simulink model "Simulink_Lin_og_NonLin"  (R2020b)
settings: Solver=VariableStepAuto  StartTime=0.0  StopTime=4  RelTol=1e-3
values from neighbouring files (symbols this model uses):
  b = 0.1    [Simulink_konstanter.m]
  g = 9.82    [Simulink_konstanter.m]
  I = 1/12    (= 0.0833333333333)    [Simulink_konstanter.m]
  Kp = 30    [Simulink_konstanter.m]
  l = 0.5    [Simulink_konstanter.m]
  m = 1    [Simulink_konstanter.m]
  Td = 1/7    (= 0.142857142857)    [Simulink_konstanter.m]
  Ti = 1    [Simulink_konstanter.m]
  u_bar = -(l*g*m*sqrt(3)) / 2    [Simulink_konstanter.m]
  y_bar = pi/3    (= 1.0471975512)    [Simulink_konstanter.m]
settings Model: Creator=madsw  LastModifiedBy=madsw

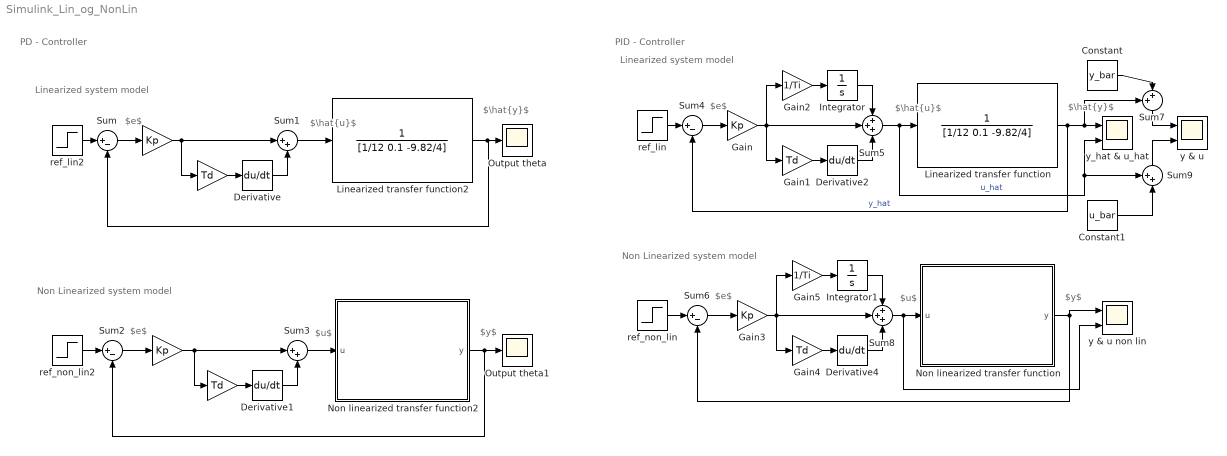
== system Simulink_Lin_og_NonLin ==
  note: PD - Controller
  note: Linearized system model
  note: Non Linearized system model
  note: $\hat{u}$
  note: $\hat{y}$
  note: $e$
  note: $u$
  note: $y$
  note: $e$
  note: Non Linearized system model
  note: $u$
  note: $y$
  note: Linearized system model
  note: $e$
  note: $\hat{u}$
  note: $\hat{y}$
  note: $e$
  note: PID - Controller
  " " : Gain  Gain=Td
  "  " : Gain  Gain=Kp
  "     " : Gain  Gain=Kp
  "              " : Gain  Gain=Td
  Constant : Constant  Value=y_bar
  Constant1 : Constant  Value=u_bar
  Derivative{,1..2,4} (4 alike) : Derivative
  Gain : Gain  Gain=Kp
  Gain1 : Gain  Gain=Td
  Gain2 : Gain  Gain=1/Ti
  Gain3 : Gain  Gain=Kp
  Gain4 : Gain  Gain=Td
  Gain5 : Gain  Gain=1/Ti
  Integrator : Integrator
  Integrator1 : Integrator
  Linearized transfer function : TransferFcn  Numerator=1  Denominator=[1/12 0.1 -9.82/4]
  Linearized transfer function2 : TransferFcn  Numerator=1  Denominator=[1/12 0.1 -9.82/4]
  Non linearized transfer function : Subsystem
  Non linearized transfer function2 : Subsystem
  Output theta : Scope
  Output theta1 : Scope
  Sum{,2,4,6} (4 alike) : Sum  Inputs=|+-
  Sum1 : Sum  Inputs=|++
  Sum3 : Sum  Inputs=|++
  Sum5 : Sum  Inputs=+++
  Sum7 : Sum  Inputs=++|
  Sum8 : Sum  Inputs=+++
  Sum9 : Sum  Inputs=++|
  ref_lin : Step  Time=0  After=pi/3  SampleTime=0
  ref_lin2 : Step  Time=0  After=pi/3  SampleTime=0
  ref_non_lin : Step  Time=0  After=pi/3  SampleTime=0
  ref_non_lin2 : Step  Time=0  After=pi/3  SampleTime=0
  y & u : Scope  NumInputPorts=2
  y & u non lin : Scope  NumInputPorts=2
  y_hat & u_hat : Scope  NumInputPorts=2
  wires:
  Linearized transfer function2/1 -> Sum/2, Output theta/1
  ref_lin2/1 -> Sum/1
  " "/1 -> Derivative/1
  Sum/1 -> "  "/1
  "  "/1 -> " "/1, Sum1/1
  Derivative/1 -> Sum1/2
  Sum1/1 -> Linearized transfer function2/1
  Sum2/1 -> "     "/1
  Derivative1/1 -> Sum3/2
  "              "/1 -> Derivative1/1
  "     "/1 -> Sum3/1, "              "/1
  Sum3/1 -> Non linearized transfer function2/1(u)
  Non linearized transfer function2/1(y) -> Sum2/2, Output theta1/1
  ref_non_lin2/1 -> Sum2/1
  ref_non_lin/1 -> Sum6/1
  Non linearized transfer function/1(y) -> y & u non lin/1, Sum6/2
  Derivative2/1 -> Sum5/3
  Gain/1 -> Gain2/1, Gain1/1, Sum5/2
  Sum5/1 -> y_hat & u_hat/2, Sum9/1, Linearized transfer function/1  "u_hat"
  Linearized transfer function/1 -> Sum7/1, y_hat & u_hat/1, Sum4/2  "y_hat"
  ref_lin/1 -> Sum4/1
  Gain2/1 -> Integrator/1
  Integrator/1 -> Sum5/1
  Sum4/1 -> Gain/1
  Gain1/1 -> Derivative2/1
  Gain3/1 -> Gain5/1, Gain4/1, Sum8/2
  Gain5/1 -> Integrator1/1
  Gain4/1 -> Derivative4/1
  Derivative4/1 -> Sum8/3
  Integrator1/1 -> Sum8/1
  Sum8/1 -> y & u non lin/2, Non linearized transfer function/1(u)
  Sum6/1 -> Gain3/1
  Constant/1 -> Sum7/2
  Sum7/1 -> y & u/1
  Constant1/1 -> Sum9/2
  Sum9/1 -> y & u/2

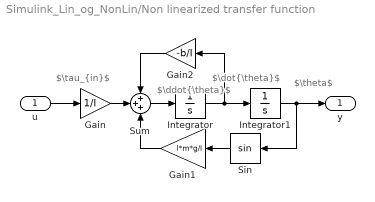
== system Simulink_Lin_og_NonLin/Non linearized transfer function ==
  note: $\ddot{\theta}$
  note: $\dot{\theta}$
  note: $\theta$
  note: $\tau_{in}$
  u : Inport
  Gain : Gain  Gain=1/I
  Gain1 : Gain  Gain=l*m*g/I
  Gain2 : Gain  Gain=-b/I
  Integrator : Integrator
  Integrator1 : Integrator
  Sin : Trigonometry
  Sum : Sum  Inputs=+++
  y : Outport
  wires:
  u/1 -> Gain/1
  Gain1/1 -> Sum/3
  Gain2/1 -> Sum/1
  Gain/1 -> Sum/2
  Sin/1 -> Gain1/1
  Sum/1 -> Integrator/1
  Integrator/1 -> Gain2/1, Integrator1/1
  Integrator1/1 -> Sin/1, y/1

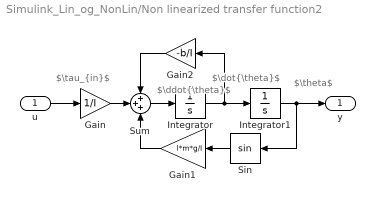
== system Simulink_Lin_og_NonLin/Non linearized transfer function2 ==
  note: $\ddot{\theta}$
  note: $\dot{\theta}$
  note: $\theta$
  note: $\tau_{in}$
  u : Inport
  Gain : Gain  Gain=1/I
  Gain1 : Gain  Gain=l*m*g/I
  Gain2 : Gain  Gain=-b/I
  Integrator : Integrator
  Integrator1 : Integrator
  Sin : Trigonometry
  Sum : Sum  Inputs=+++
  y : Outport
  wires:
  u/1 -> Gain/1
  Gain1/1 -> Sum/3
  Gain2/1 -> Sum/1
  Gain/1 -> Sum/2
  Sin/1 -> Gain1/1
  Sum/1 -> Integrator/1
  Integrator/1 -> Gain2/1, Integrator1/1
  Integrator1/1 -> Sin/1, y/1
